simulink model "sim_VSS_steady_degenerate_motion"  (R2019a)
settings: Solver=FixedStepAuto  StartTime=0.0  StopTime=end_time  FixedStep=FStep  RelTol=1e-3  EnableMultiTasking=on
undefined symbols (not defined in the file): h, k, K, p, T, x0, y0
libraries: simulink_extras x1
settings Model: Creator=user  LastModifiedBy=ogure
settings SolverCC: SolverResetMethod=Robust
settings DataIOCC: LimitDataPoints=on  SaveFormat=Array  SaveOutput=off  ReturnWorkspaceOutputs=off  OutputSaveName=X,X4,L,H
settings OptimizationCC: LifeSpan=inf
settings DebuggingCC: SolverPrmCheckMsg=warning  SFUnexpectedBacktrackingDiag=warning  SFNoUnconditionalDefaultTransitionDiag=warning  SFExecutionAtInitializationDiag=none  ArithmeticOperatorsInVariantConditions=warning
settings HardwareCC: ProdBitPerPointer=32  ProdBitPerSizeT=32  ProdBitPerPtrDiffT=32  ProdLargestAtomicFloat=None  ProdIntDivRoundTo=Undefined  ProdEndianess=Unspecified  ProdWordSize=32  ProdHWDeviceType=32-bit Generic
settings ModelReferenceCC: PropagateSignalLabelsOutOfModel=off
settings SFSimCC: SimUseLocalCustomCode=off
settings RTWCC: RTWUseLocalCustomCode=off
settings CodeAppCC: StateflowObjectComments=on
settings GRTTargetCC: TargetLangStandard=C89/C90 (ANSI)  GeneratePreprocessorConditionals=Disable all
settings ConfigComp: CovMetricSettings=dw  CovHtmlReporting=on  CovSaveCumulativeToWorkspaceVar=on  CovSaveSingleToWorkspaceVar=on  CovExternalEMLEnable=off  CovSFcnEnable=off

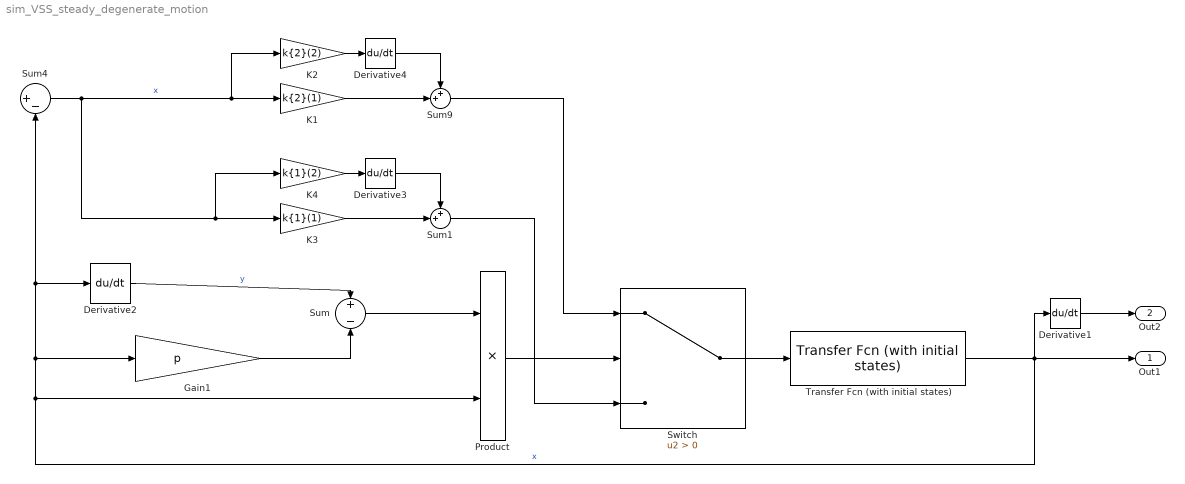
== system sim_VSS_steady_degenerate_motion ==
  Derivative{1..4} (4 alike) : Derivative  CoefficientInTFapproximation=0.00000001
  Gain1 : Gain  Gain=p
  K1 : Gain  Gain=k{2}(1)
  K2 : Gain  Gain=k{2}(2)
  K3 : Gain  Gain=k{1}(1)
  K4 : Gain  Gain=k{1}(2)
  Product : Product
  Sum : Sum  Inputs=+-
  Sum1 : Sum  Inputs=++|
  Sum4 : Sum  Inputs=|+-
  Sum9 : Sum  Inputs=++|
  Switch : Switch  Criteria=u2 > Threshold  ZeroCross=off
  Transfer Fcn (with initial states) : simulink_extras/Additional Linear/Transfer Fcn (with initial states)  N=[K]  D="[ T^2  2*T*h  1]"  X0=[x0, y0]
  Out1 : Outport  SignalName=x
  Out2 : Outport  Port=2  SignalName=y
  wires:
  Switch/1 -> Transfer Fcn (with initial states)/1
  Gain1/1 -> Sum/2
  Derivative2/1 -> Sum/1  "y"
  Product/1 -> Switch/2
  Sum/1 -> Product/1
  Derivative1/1 -> Out2/1
  Transfer Fcn (with initial states)/1 -> Product/2, Sum4/2, Derivative2/1, Gain1/1, Derivative1/1, Out1/1  "x"
  K1/1 -> Sum9/2
  K2/1 -> Derivative4/1
  Derivative4/1 -> Sum9/1
  Sum9/1 -> Switch/1
  K4/1 -> Derivative3/1
  Derivative3/1 -> Sum1/1
  K3/1 -> Sum1/2
  Sum4/1 -> K4/1, K3/1, K1/1, K2/1  "x"
  Sum1/1 -> Switch/3
